simulink model "digitaltwins"  (R2020b)
settings: Solver=ode4  StartTime=0.0  StopTime=30  FixedStep=0.01  RelTol=1e-3
libraries: simulink x2
settings Model: Creator=skets  LastModifiedBy=PC
settings SolverCC: ConcurrentTasks=on  PositivePriorityOrder=on
settings DataIOCC: ReturnWorkspaceOutputs=off
settings OptimizationCC: BlockReduction=off  OptimizeBlockIOStorage=off
settings DebuggingCC: ArithmeticOperatorsInVariantConditions=warning
settings HardwareCC: ProdBitPerLong=64  ProdLongLongMode=on  ProdHWDeviceType=Intel->x86-64 (Linux 64)
settings SFSimCC: SimUseLocalCustomCode=off  CustomCodeUndefinedFunction=UseInterfaceOnly
settings RTWCC: Description=Simulink Real-Time  SystemTargetFile=slrealtime.tlc  TemplateMakefile=slrealtime_default_tmf  RTWUseLocalCustomCode=off  Toolchain=Simulink Real-Time Toolchain  BuildConfiguration=Faster Runs  CodeExecutionProfiling=on  TargetLang=C++

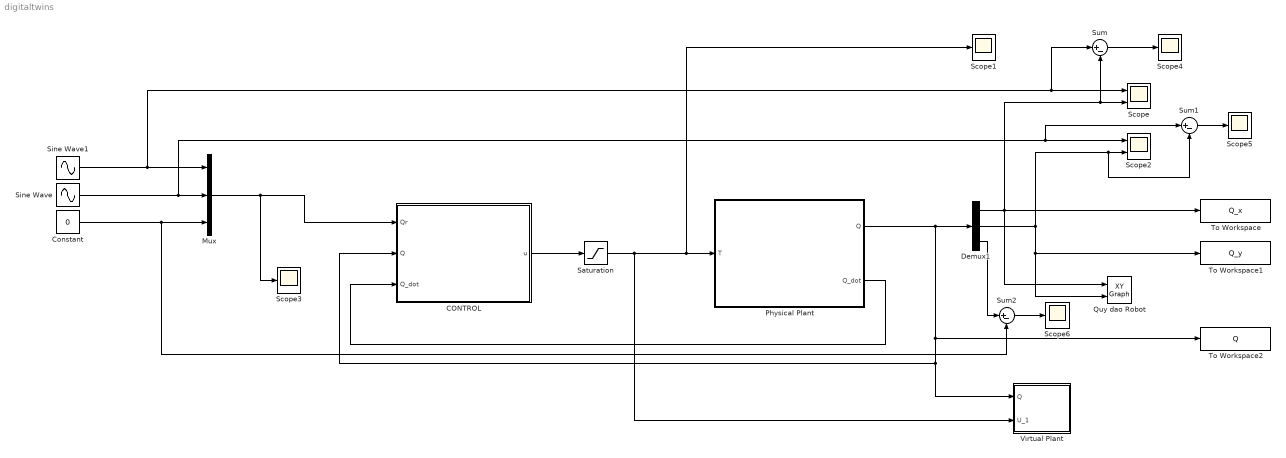
== system digitaltwins ==
  CONTROL : Subsystem
  Constant : Constant  Value=0
  Demux1 : Demux  Outputs=3
  Mux : Mux  Inputs=3
  Physical Plant : Subsystem
  Quy dao Robot : simulink/Sinks/XY Graph  xmin=0  xmax=5  ymin=0  ymax=5  st=-1
  Saturation : Saturate  UpperLimit=10  LowerLimit=-10
  Scope : Scope  NumInputPorts=2
  Scope{1,3..6} (5 alike) : Scope
  Scope2 : Scope  NumInputPorts=2
  Sine Wave : Sin  Bias=3  Frequency=4*pi/15
  Sine Wave1 : Sin  Bias=2.5  Frequency=2*pi/15
  Sum : Sum  Inputs=|+-
  Sum1 : Sum  Inputs=|+-
  Sum2 : Sum  Inputs=|+-
  To Workspace : ToWorkspace  VariableName=Q_x  SaveFormat=Timeseries  SampleTime=-1
  To Workspace1 : ToWorkspace  VariableName=Q_y  SaveFormat=Timeseries  SampleTime=-1
  To Workspace2 : ToWorkspace  VariableName=Q  SaveFormat=Timeseries  SampleTime=-1
  Virtual Plant : Subsystem
  wires:
  CONTROL/1(u) -> Saturation/1
  Physical Plant/2(Q_dot) -> CONTROL/3(Q_dot)
  Physical Plant/1(Q) -> Virtual Plant/1(Q), CONTROL/2(Q), To Workspace2/1, Demux1/1
  Demux1/1 -> Sum/2, Scope/2, To Workspace/1, Quy dao Robot/1
  Demux1/2 -> Sum1/2, Scope2/2, Quy dao Robot/2, To Workspace1/1
  Mux/1 -> Scope3/1, CONTROL/1(Qr)
  Sine Wave1/1 -> Sum/1, Scope/1, Mux/1
  Sine Wave/1 -> Sum1/1, Scope2/1, Mux/2
  Constant/1 -> Sum2/2, Mux/3
  Sum/1 -> Scope4/1
  Sum1/1 -> Scope5/1
  Demux1/3 -> Sum2/1
  Sum2/1 -> Scope6/1
  Saturation/1 -> Virtual Plant/2(U_1), Scope1/1, Physical Plant/1(T)

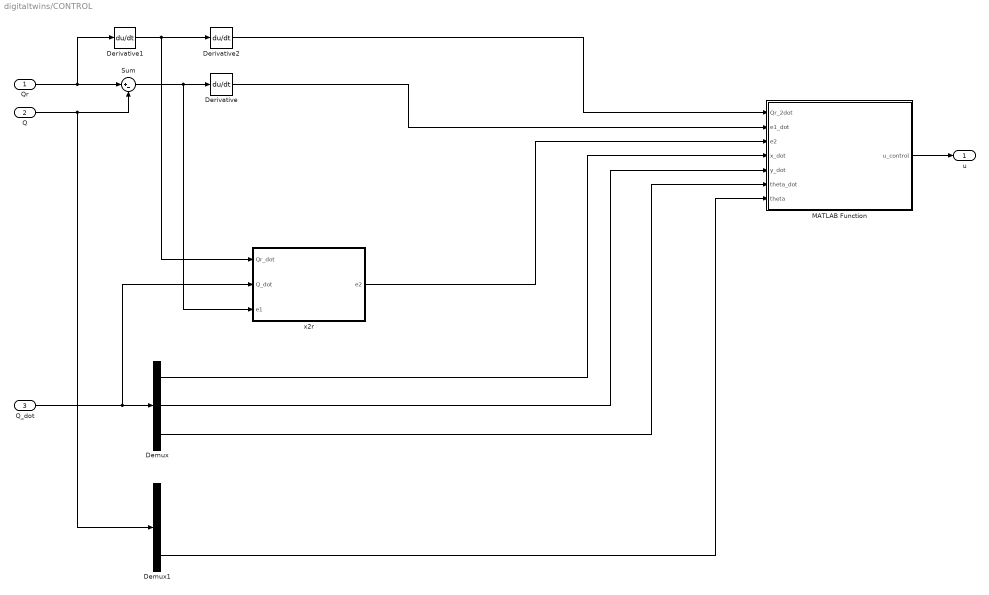
== system digitaltwins/CONTROL ==
  Qr : Inport
  Q : Inport  Port=2  PortDimensions=3
  Q_dot : Inport  Port=3
  Demux : Demux  Outputs=3
  Demux1 : Demux  Outputs=3
  Derivative : Derivative
  Derivative1 : Derivative
  Derivative2 : Derivative
  MATLAB Function : MATLAB Function  TreatAsAtomicUnit=on
  Sum : Sum  Inputs=|+-
  x2r : MATLAB Function  TreatAsAtomicUnit=on
  u : Outport  VectorParamsAs1DForOutWhenUnconnected=off
  wires:
  Qr/1 -> Derivative1/1, Sum/1
  Derivative1/1 -> x2r/1(Qr_dot), Derivative2/1
  MATLAB Function/1(u_control) -> u/1
  Q/1 -> Sum/2, Demux1/1
  Q_dot/1 -> x2r/2(Q_dot), Demux/1
  Demux/1 -> MATLAB Function/4(x_dot)
  Demux/2 -> MATLAB Function/5(y_dot)
  Demux/3 -> MATLAB Function/6(theta_dot)
  Demux1/3 -> MATLAB Function/7(theta)
  Sum/1 -> x2r/3(e1), Derivative/1
  Derivative2/1 -> MATLAB Function/1(Qr_2dot)
  Derivative/1 -> MATLAB Function/2(e1_dot)
  x2r/1(e2) -> MATLAB Function/3(e2)

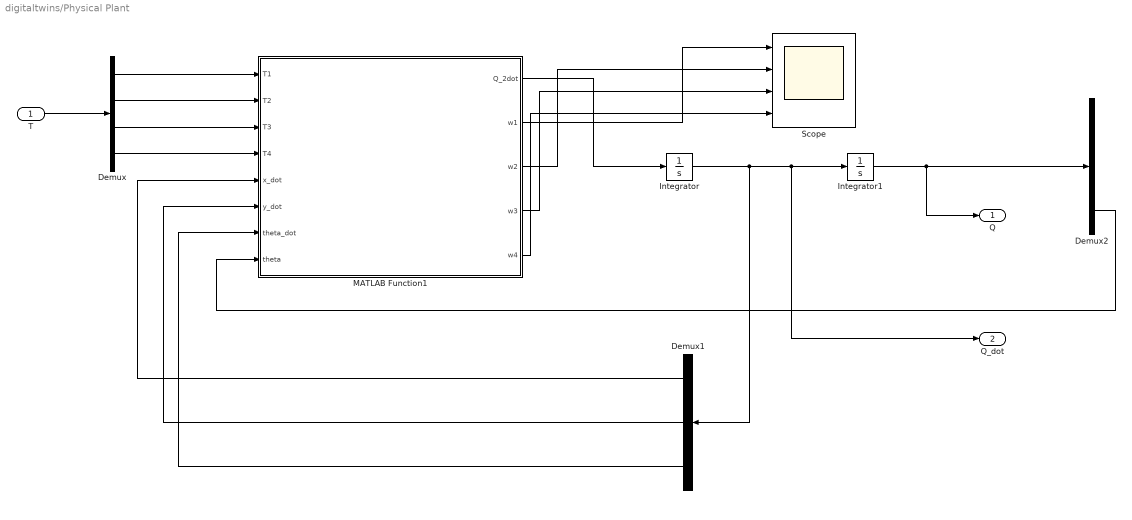
== system digitaltwins/Physical Plant ==
  T : Inport  PortDimensions=4
  Demux : Demux
  Demux1 : Demux  Outputs=3
  Demux2 : Demux  Outputs=3
  Integrator : Integrator
  Integrator1 : Integrator  InitialCondition=[2.5 3 0]
  MATLAB Function1 : MATLAB Function  TreatAsAtomicUnit=on
  Scope : Scope  NumInputPorts=4
  Q : Outport  VectorParamsAs1DForOutWhenUnconnected=off
  Q_dot : Outport  Port=2  VectorParamsAs1DForOutWhenUnconnected=off
  wires:
  Demux/1 -> MATLAB Function1/1(T1)
  Demux/2 -> MATLAB Function1/2(T2)
  Demux/3 -> MATLAB Function1/3(T3)
  Demux/4 -> MATLAB Function1/4(T4)
  MATLAB Function1/1(Q_2dot) -> Integrator/1
  Integrator/1 -> Q_dot/1, Integrator1/1, Demux1/1
  Demux1/1 -> MATLAB Function1/5(x_dot)
  Demux1/2 -> MATLAB Function1/6(y_dot)
  Demux1/3 -> MATLAB Function1/7(theta_dot)
  Integrator1/1 -> Demux2/1, Q/1
  Demux2/3 -> MATLAB Function1/8(theta)
  T/1 -> Demux/1
  MATLAB Function1/2(w1) -> Scope/1
  MATLAB Function1/3(w2) -> Scope/2
  MATLAB Function1/4(w3) -> Scope/3
  MATLAB Function1/5(w4) -> Scope/4

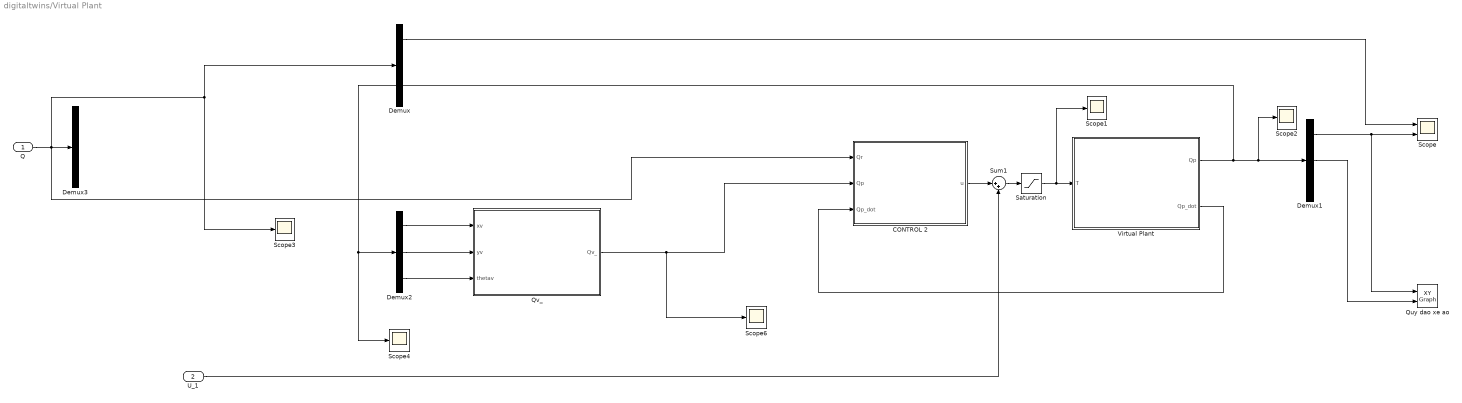
== system digitaltwins/Virtual Plant ==
  Q : Inport
  U_1 : Inport  Port=2
  CONTROL 2 : Subsystem
  Demux{,1..3} (4 alike) : Demux  Outputs=3
  Quy dao xe ao : simulink/Sinks/XY Graph  xmin=0  xmax=5  ymin=0  ymax=5  st=-1
  Qv_ : MATLAB Function  TreatAsAtomicUnit=on
  Saturation : Saturate  UpperLimit=10  LowerLimit=-10
  Scope : Scope  NumInputPorts=2
  Scope{1..4,6} (5 alike) : Scope
  Sum1 : Sum  Inputs=|++
  Virtual Plant : Subsystem
  wires:
  Demux/1 -> Scope/1
  Virtual Plant/1(Qp) -> Demux2/1, Scope4/1, Scope2/1, Demux1/1
  Virtual Plant/2(Qp_dot) -> CONTROL 2/3(Qp_dot)
  Demux2/1 -> Qv_/1(xv)
  Demux2/2 -> Qv_/2(yv)
  Demux2/3 -> Qv_/3(thetav)
  Qv_/1(Qv_) -> Scope6/1, CONTROL 2/2(Qp)
  Demux1/1 -> Quy dao xe ao/1, Scope/2
  Demux1/2 -> Quy dao xe ao/2
  Q/1 -> CONTROL 2/1(Qr), Scope3/1, Demux/1, Demux3/1
  U_1/1 -> Sum1/2
  Sum1/1 -> Saturation/1
  CONTROL 2/1(u) -> Sum1/1
  Saturation/1 -> Scope1/1, Virtual Plant/1(T)

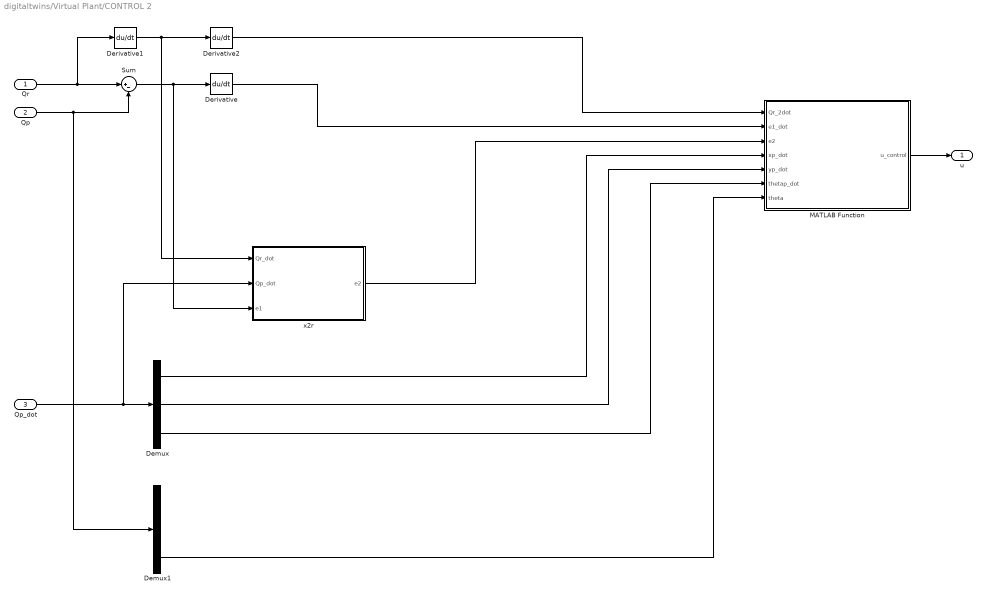
== system digitaltwins/Virtual Plant/CONTROL 2 ==
  Qr : Inport
  Qp : Inport  Port=2  PortDimensions=3
  Qp_dot : Inport  Port=3  PortDimensions=3
  Demux : Demux  Outputs=3
  Demux1 : Demux  Outputs=3
  Derivative : Derivative
  Derivative1 : Derivative
  Derivative2 : Derivative
  MATLAB Function : MATLAB Function  TreatAsAtomicUnit=on
  Sum : Sum  Inputs=|+-
  x2r : MATLAB Function  TreatAsAtomicUnit=on
  u : Outport  VectorParamsAs1DForOutWhenUnconnected=off
  wires:
  Qr/1 -> Derivative1/1, Sum/1
  Derivative1/1 -> x2r/1(Qr_dot), Derivative2/1
  MATLAB Function/1(u_control) -> u/1
  Qp/1 -> Sum/2, Demux1/1
  Qp_dot/1 -> x2r/2(Qp_dot), Demux/1
  Demux/1 -> MATLAB Function/4(xp_dot)
  Demux/2 -> MATLAB Function/5(yp_dot)
  Demux/3 -> MATLAB Function/6(thetap_dot)
  Demux1/3 -> MATLAB Function/7(theta)
  Sum/1 -> x2r/3(e1), Derivative/1
  x2r/1(e2) -> MATLAB Function/3(e2)
  Derivative2/1 -> MATLAB Function/1(Qr_2dot)
  Derivative/1 -> MATLAB Function/2(e1_dot)

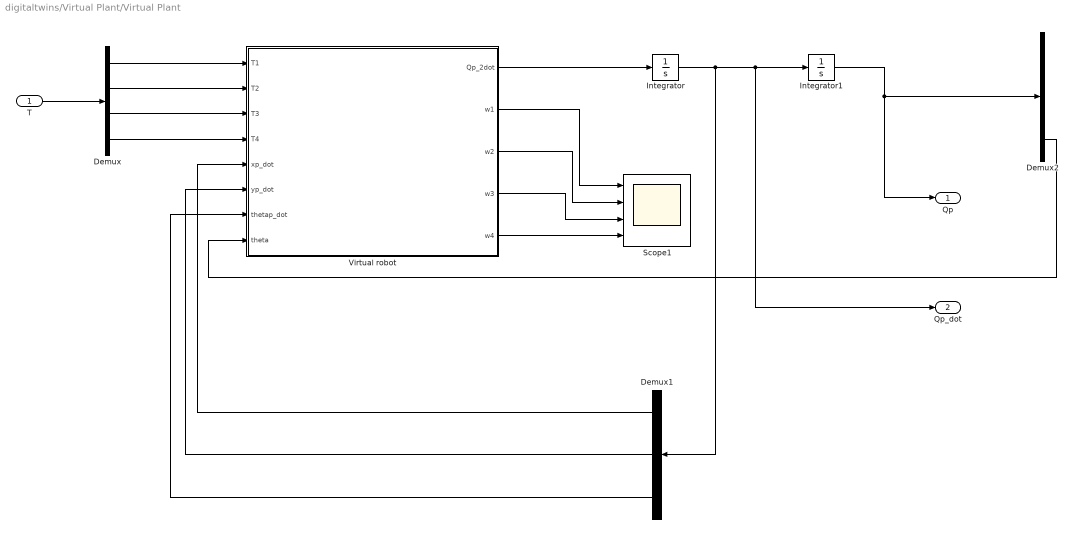
== system digitaltwins/Virtual Plant/Virtual Plant ==
  T : Inport  PortDimensions=4
  Demux : Demux
  Demux1 : Demux  Outputs=3
  Demux2 : Demux  Outputs=3
  Integrator : Integrator
  Integrator1 : Integrator  InitialCondition=[2.5 3 0]
  Scope1 : Scope  NumInputPorts=4
  Virtual robot : MATLAB Function  TreatAsAtomicUnit=on
  Qp : Outport  VectorParamsAs1DForOutWhenUnconnected=off
  Qp_dot : Outport  Port=2  VectorParamsAs1DForOutWhenUnconnected=off
  wires:
  Demux/1 -> Virtual robot/1(T1)
  Demux/2 -> Virtual robot/2(T2)
  Demux/3 -> Virtual robot/3(T3)
  Demux/4 -> Virtual robot/4(T4)
  Virtual robot/1(Qp_2dot) -> Integrator/1
  Integrator/1 -> Demux1/1, Qp_dot/1, Integrator1/1
  Demux1/1 -> Virtual robot/5(xp_dot)
  Demux1/2 -> Virtual robot/6(yp_dot)
  Demux1/3 -> Virtual robot/7(thetap_dot)
  Integrator1/1 -> Demux2/1, Qp/1
  Demux2/3 -> Virtual robot/8(theta)
  T/1 -> Demux/1
  Virtual robot/2(w1) -> Scope1/1
  Virtual robot/3(w2) -> Scope1/2
  Virtual robot/4(w3) -> Scope1/3
  Virtual robot/5(w4) -> Scope1/4

== matlab function digitaltwins/Virtual Plant/CONTROL 2/x2r ==
  data: Qr_dot input; Qp_dot input; e2 output; e1 input
function e2  = fcn(Qr_dot,Qp_dot,e1)

k1 = [10 0 0;
      0 10 0;
      0 0 10];
 
%x2r_dot = (Qr_2dot+k1*e1_dot);
x2r = Qr_dot + k1*e1;
e2 = x2r - Qp_dot;

== matlab function digitaltwins/Physical Plant/MATLAB Function1 ==
  data: T1 input; Q_2dot output; T2 input; T3 input; T4 input; x_dot input; y_dot input; theta_dot input; theta input; w1 output; w2 output; w3 output; w4 output
function [Q_2dot,w1,w2,w3,w4] = fcn(T1, T2, T3, T4,x_dot,y_dot,theta_dot,theta)
m=5;
I=5;
Ib=0.1;
l1= 0.3;
l2=0.3;
r=0.097/2;
g=9.81;
u=0.01;
N = m*g/4;
M=[(m+4*Ib/(r*r)) 0 0; 0 (m+4*Ib/(r*r)) 0; 0 0 (I+4*Ib*(l1+l2)*(l1+l2)/(r*r))];
C= [(m+4*Ib/(r*r))*y_dot*theta_dot;-(m+4*Ib/(r*r))*x_dot*theta_dot;0 ];
B=(1/r)*[(cos(theta)+sin(theta)) (cos(theta)-sin(theta)) (cos(theta)+sin(theta)) (cos(theta)-sin(theta));
         (-cos(theta)+sin(theta)) (cos(theta)+sin(theta)) (-cos(theta)+sin(theta)) (cos(theta)+sin(theta)); 
         (-(l1+l2)) (l1+l2) (l1+l2) (-(l1+l2)) ];
T=[T1;T2;T3;T4];
xm= cos(theta)*x_dot+sin(theta)*y_dot;
ym= -sin(theta)*x_dot+cos(theta)*y_dot;
w1 = (1/r)*(xm-ym-(l1+l2)*theta_dot);
w2 = (1/r)*(xm+ym+(l1+l2)*theta_dot);
w3 = (1/r)*(xm-ym+(l1+l2)*theta_dot);
w4 = (1/r)*(xm+ym-(l1+l2)*theta_dot);
w_max = 2*pi;
if w1 > w_max
    w1 = w_max;
elseif w1 < -w_max
    w1 = -w_max;
end
if w2 > w_max
    w2 = w_max;
elseif w2 < -w_max
    w2 = -w_max;
end
if w3 > w_max
    w3 = w_max;
elseif w3 < -w_max
    w3 = -w_max;
end
if w4 > w_max
    w4 = w_max;
elseif w4 < -w_max
    w4 = -w_max;
end
Xi=[u*r*N*sign(w1);u*r*N*sign(w2);u*r*N*sign(w3);u*N*r*sign(w4)];

Q_2dot=inv(M)*(B*T-C-B*Xi);

== matlab function digitaltwins/CONTROL/MATLAB Function ==
  data: Qr_2dot input; u_control output; e1_dot input; e2 input; x_dot input; y_dot input; theta_dot input; theta input
function u_control = fcn(Qr_2dot,e1_dot,e2,x_dot,y_dot,theta_dot,theta)

m=5;
I=5;
Ib=0.1;
l1= 0.3;
l2=0.3;
r=0.097/2;
g=9.81;
u=0.01;
N = m*g/4;
M=[(m+4*Ib/(r*r)) 0 0; 0 (m+4*Ib/(r*r)) 0; 0 0 (I+4*Ib*(l1+l2)*(l1+l2)/(r*r))];
C= [(m+4*Ib/(r*r))*y_dot*theta_dot;-(m+4*Ib/(r*r))*x_dot*theta_dot;0 ];
B=(1/r)*[(cos(theta)+sin(theta)) (cos(theta)-sin(theta)) (cos(theta)+sin(theta)) (cos(theta)-sin(theta));
    (-cos(theta)+sin(theta)) (cos(theta)+sin(theta)) (-cos(theta)+sin(theta)) (cos(theta)+sin(theta)); 
    (-(l1+l2)) (l1+l2) (l1+l2) (-(l1+l2)) ];

xm= cos(theta)*x_dot+sin(theta)*y_dot;
ym= -sin(theta)*x_dot+cos(theta)*y_dot;
w1 = (1/r)*(xm-ym-(l1+l2)*theta_dot);
w2 = (1/r)*(xm+ym+(l1+l2)*theta_dot);
w3 = (1/r)*(xm-ym+(l1+l2)*theta_dot);
w4 = (1/r)*(xm+ym-(l1+l2)*theta_dot);
w_max = 2*pi;
if w1 > w_max
    w1 = w_max;
elseif w1 < -w_max
    w1 = -w_max;
end
if w2 > w_max
    w2 = w_max;
elseif w2 < -w_max
    w2 = -w_max;
end
if w3 > w_max
    w3 = w_max;
elseif w3 < -w_max
    w3 = -w_max;
end
if w4 > w_max
    w4 = w_max;
elseif w4 < -w_max
    w4 = -w_max;
end
Xi=[u*r*N*sign(w1);u*r*N*sign(w2);u*r*N*sign(w3);u*N*r*sign(w4)];

k1 = [4 0 0;
      0 4 0;
      0 0 4];
k2 = [4 0 0;
      0 4 0;
      0 0 4];
  
u_control = B'*inv(B*B')*M*((Qr_2dot+k1*e1_dot)+inv(M)*C+inv(M)*B*Xi+k2*e2);

== matlab function digitaltwins/CONTROL/x2r ==
  data: Qr_dot input; Q_dot input; e2 output; e1 input
function e2  = fcn(Qr_dot,Q_dot,e1)

k1 = [4 0 0;
      0 4 0;
      0 0 4];
 
%x2r_dot = (Qr_2dot+k1*e1_dot);
x2r = Qr_dot + k1*e1;
e2 = x2r - Q_dot;

== matlab function digitaltwins/Virtual Plant/Qv_ ==
  data: Qv_ output; xv input; yv input; thetav input
function Qv_ = fcn(xv, yv,thetav)

xp_t0 = 2;
yp_t0 = 2;
thetap_t0 = 0;
xv_t0 = 2;
yv_t0 = 2;
thetav_t0 = 0;
delta_theta = thetap_t0 - thetav_t0;
delta_x = xp_t0 - xv_t0*cos(delta_theta) - yv_t0*sin(delta_theta);
delta_y = yp_t0 - xv_t0*sin(delta_theta) - yv_t0*cos(delta_theta);

T_delta = [ 1 0 0 delta_x;
            0 1 0 delta_y;
            0 0 1 delta_theta;
            0 0 0 1];
R_delta = [ cos(delta_theta) -sin(delta_theta) 0 0;
            sin(delta_theta) cos(delta_theta) 0 0;
            0 0 1 0;
            0 0 0 1 ];   
H = T_delta*R_delta;
Qv_temp = H*[ xv; yv; thetav; 1];
Qv_ = [Qv_temp(1);Qv_temp(2);Qv_temp(3)];

== matlab function digitaltwins/Virtual Plant/Virtual Plant/Virtual robot ==
  data: T1 input; Qp_2dot output; T2 input; T3 input; T4 input; xp_dot input; yp_dot input; thetap_dot input; theta input; w1 output; w2 output; w3 output; w4 output
function [Qp_2dot,w1,w2,w3,w4]  = fcn(T1, T2, T3, T4,xp_dot,yp_dot,thetap_dot,theta)
m=5;
I=5;
Ib=0.1;
l1= 0.3;
l2=0.3;
r=0.097/2;
g=9.81;
u=0.01;
N = m*g/4;
M=[(m+4*Ib/(r*r)) 0 0; 0 (m+4*Ib/(r*r)) 0; 0 0 (I+4*Ib*(l1+l2)*(l1+l2)/(r*r))];
C= [(m+4*Ib/(r*r))*yp_dot*thetap_dot;-(m+4*Ib/(r*r))*xp_dot*thetap_dot;0 ];
B=(1/r)*[(cos(theta)+sin(theta)) (cos(theta)-sin(theta)) (cos(theta)+sin(theta)) (cos(theta)-sin(theta));
         (-cos(theta)+sin(theta)) (cos(theta)+sin(theta)) (-cos(theta)+sin(theta)) (cos(theta)+sin(theta)); 
         (-(l1+l2)) (l1+l2) (l1+l2) (-(l1+l2)) ];
T=[T1;T2;T3;T4];
xm= cos(theta)*xp_dot+sin(theta)*yp_dot;
ym= -sin(theta)*xp_dot+cos(theta)*yp_dot;
w1 = (1/r)*(xm-ym-(l1+l2)*thetap_dot);
w2 = (1/r)*(xm+ym+(l1+l2)*thetap_dot);
w3 = (1/r)*(xm-ym+(l1+l2)*thetap_dot);
w4 = (1/r)*(xm+ym-(l1+l2)*thetap_dot);
w_max = 2*pi;
if w1 > w_max
    w1 = w_max;
elseif w1 < -w_max
    w1 = -w_max;
end
if w2 > w_max
    w2 = w_max;
elseif w2 < -w_max
    w2 = -w_max;
end
if w3 > w_max
    w3 = w_max;
elseif w3 < -w_max
    w3 = -w_max;
end
if w4 > w_max
    w4 = w_max;
elseif w4 < -w_max
    w4 = -w_max;
end
Xi=[u*r*N*sign(w1);u*r*N*sign(w2);u*r*N*sign(w3);u*N*r*sign(w4)];

Qp_2dot=inv(M)*(B*T-C-B*Xi);

== matlab function digitaltwins/Virtual Plant/CONTROL 2/MATLAB Function ==
  data: Qr_2dot input; u_control output; e1_dot input; e2 input; xp_dot input; yp_dot input; thetap_dot input; theta input
function u_control = fcn(Qr_2dot,e1_dot,e2,xp_dot,yp_dot,thetap_dot,theta)

m=5;
I=5;
Ib=0.1;
l1= 0.3;
l2=0.3;
r=0.097/2;
g=9.81;
u=0.01;
N = m*g/4;
M=[(m+4*Ib/(r*r)) 0 0; 0 (m+4*Ib/(r*r)) 0; 0 0 (I+4*Ib*(l1+l2)*(l1+l2)/(r*r))];
C= [(m+4*Ib/(r*r))*yp_dot*thetap_dot;-(m+4*Ib/(r*r))*xp_dot*thetap_dot;0 ];
B=(1/r)*[(cos(theta)+sin(theta)) (cos(theta)-sin(theta)) (cos(theta)+sin(theta)) (cos(theta)-sin(theta));
    (-cos(theta)+sin(theta)) (cos(theta)+sin(theta)) (-cos(theta)+sin(theta)) (cos(theta)+sin(theta)); 
    (-(l1+l2)) (l1+l2) (l1+l2) (-(l1+l2)) ];

xm= cos(theta)*xp_dot+sin(theta)*yp_dot;
ym= -sin(theta)*xp_dot+cos(theta)*yp_dot;
w1 = (1/r)*(xm-ym-(l1+l2)*thetap_dot);
w2 = (1/r)*(xm+ym+(l1+l2)*thetap_dot);
w3 = (1/r)*(xm-ym+(l1+l2)*thetap_dot);
w4 = (1/r)*(xm+ym-(l1+l2)*thetap_dot);
w_max = 2*pi;
if w1 > w_max
    w1 = w_max;
elseif w1 < -w_max
    w1 = -w_max;
end
if w2 > w_max
    w2 = w_max;
elseif w2 < -w_max
    w2 = -w_max;
end
if w3 > w_max
    w3 = w_max;
elseif w3 < -w_max
    w3 = -w_max;
end
if w4 > w_max
    w4 = w_max;
elseif w4 < -w_max
    w4 = -w_max;
end
Xi=[u*r*N*sign(w1);u*r*N*sign(w2);u*r*N*sign(w3);u*N*r*sign(w4)];

k1 = [10 0 0;
      0 10 0;
      0 0 10];
k2 = [10 0 0;
      0 10 0;
      0 0 10];
  
u_control = B'*inv(B*B')*M*((Qr_2dot+k1*e1_dot)+inv(M)*C+inv(M)*B*Xi+k2*e2);
